simulink model "Dynamics"  (R2022b)
settings: Solver=FixedStepAuto  StartTime=0.0  StopTime=10  FixedStep=0.01  RelTol=1e-3
undefined symbols (not defined in the file or in its folder): params, r, v
settings Model: Creator=lulav  LastModifiedBy=lulav
settings DataIOCC: SaveOutput=off  SaveTime=off
settings ModelReferenceCC: ModelReferenceMinAlgLoopOccurrences=on
settings GRTTargetCC: CombineOutputUpdateFcns=off

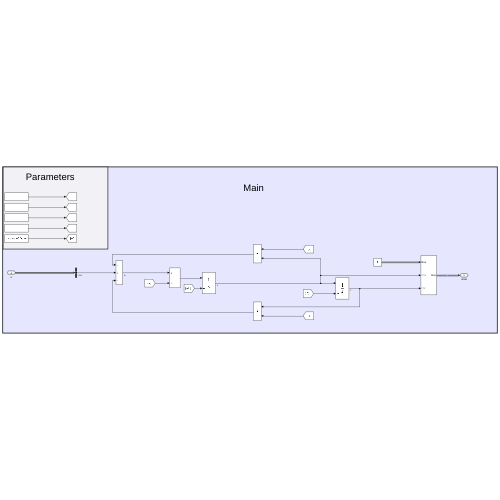
[thumbnail: Simulink's stored preview of the top-level diagram]
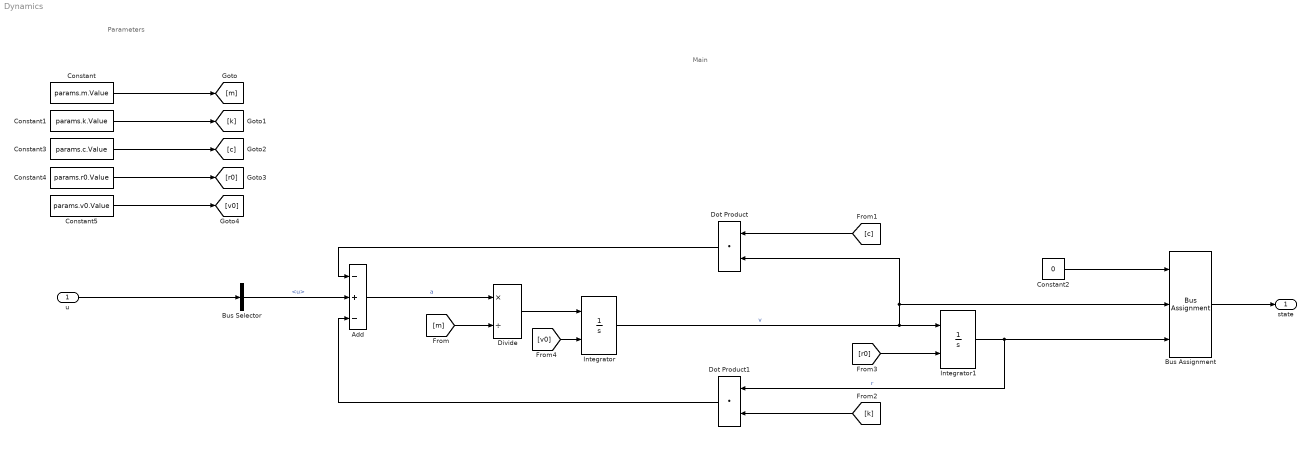
== system Dynamics ==
  note: Main
  note: Parameters
  u : Inport  OutDataTypeStr=Bus: B_Controller  PortDimensions=1  SampleTime=0  BusOutputAsStruct=on
  Add : Sum  Inputs=-+-
  Bus Assignment : BusAssignment  AssignedSignals=v,r
  Bus Selector : BusSelector  OutputSignals=u
  Constant : Constant  Value=params.m.Value
  Constant1 : Constant  Value=params.k.Value
  Constant2 : Constant  Value=0  OutDataTypeStr=Bus: B_Dynamics
  Constant3 : Constant  Value=params.c.Value
  Constant4 : Constant  Value=params.r0.Value
  Constant5 : Constant  Value=params.v0.Value
  Divide : Product  Inputs=*/
  Dot Product : DotProduct  OutDataTypeStr=Inherit: Inherit via internal rule
  Dot Product1 : DotProduct  OutDataTypeStr=Inherit: Inherit via internal rule
  Integrator : Integrator  InitialConditionSource=external
  Integrator1 : Integrator  InitialConditionSource=external
  state : Outport  OutDataTypeStr=Bus: B_Dynamics  PortDimensions=1  SampleTime=0  BusOutputAsStruct=on
  wires:
  Constant5/1 -> [v0]
  Dot Product1/1 -> Add/3
  Divide/1 -> Integrator/1
  Constant4/1 -> [r0]
  Bus Assignment/1 -> state/1
  [r0] -> Integrator1/2
  Integrator/1 -> Bus Assignment/2, Dot Product/2, Integrator1/1  "v"
  Add/1 -> Divide/1  "a"
  Constant2/1 -> Bus Assignment/1
  [c] -> Dot Product/1
  Integrator1/1 -> Bus Assignment/3, Dot Product1/1  "r"
  Constant3/1 -> [c]
  [v0] -> Integrator/2
  [k] -> Dot Product1/2
  Dot Product/1 -> Add/1
  Constant/1 -> [m]
  Constant1/1 -> [k]
  u/1 -> Bus Selector/1
  [m] -> Divide/2
  Bus Selector/1 -> Add/2  "<u>"
